simulink model "testing_discrete_tf"  (R2015b)
settings: Solver=ode23t  StartTime=0.0  StopTime=10.0  RelTol=1e-3
values from neighbouring files (symbols this model uses):
  tfa = dis_num_c2{1,1}(1)    [compensator_design.m]
  tfb = dis_num_c2{1,1}(2)    [compensator_design.m]
  tfc = dis_num_c2{1,1}(3)    [compensator_design.m]
  tfd = dis_den_c2{1,1}(1)    [compensator_design.m]
  tfe = dis_den_c2{1,1}(2)    [compensator_design.m]
  tff = dis_den_c2{1,1}(3)    [compensator_design.m]
undefined symbols (not defined in the file or in its folder): dis_den_c2, dis_num_c2
settings Model: Creator=Akshay  LastModifiedBy=Akshay

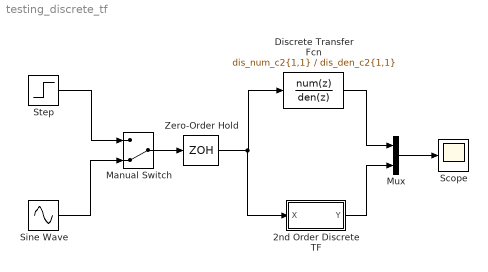
== system testing_discrete_tf ==
  2nd Order Discrete TF : Subsystem
  Discrete Transfer Fcn : DiscreteTransferFcn  Numerator=dis_num_c2{1,1}  Denominator=dis_den_c2{1,1}
  Manual Switch : ManualSwitch  CurrentSetting=0
  Mux : Mux  Inputs=2
  Scope : Scope
  Sine Wave : Sin  SampleTime=0
  Step : Step  SampleTime=0
  Zero-Order Hold : ZeroOrderHold  SampleTime=1e-5
  wires:
  Step/1 -> Manual Switch/1
  Sine Wave/1 -> Manual Switch/2
  Discrete Transfer Fcn/1 -> Mux/1
  2nd Order Discrete TF/1(Y) -> Mux/2
  Mux/1 -> Scope/1
  Manual Switch/1 -> Zero-Order Hold/1
  Zero-Order Hold/1 -> 2nd Order Discrete TF/1(X), Discrete Transfer Fcn/1

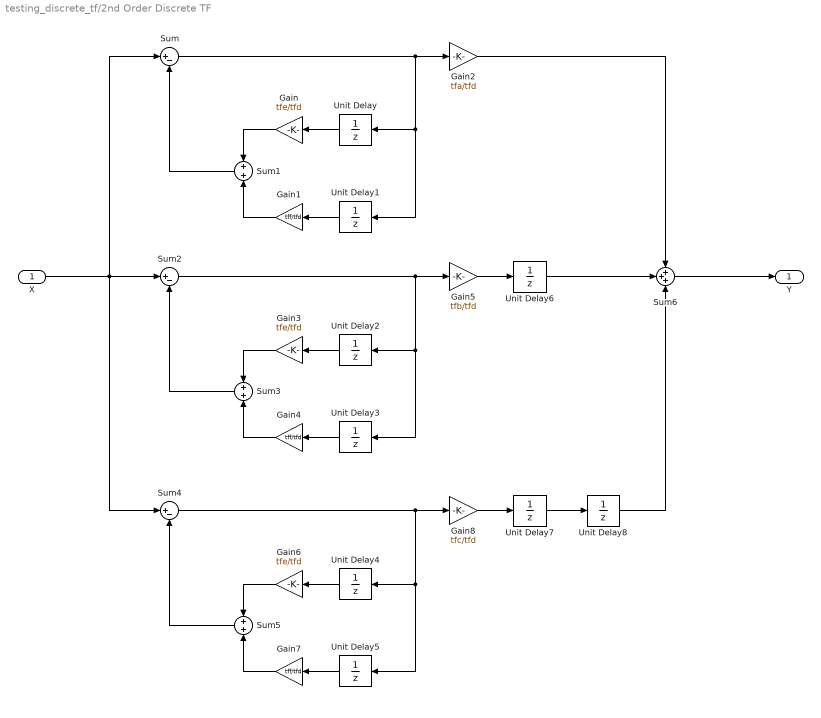
== system testing_discrete_tf/2nd Order Discrete TF ==
  X : Inport
  Gain : Gain  Gain=tfe/tfd
  Gain1 : Gain  Gain=tff/tfd
  Gain2 : Gain  Gain=tfa/tfd
  Gain3 : Gain  Gain=tfe/tfd
  Gain4 : Gain  Gain=tff/tfd
  Gain5 : Gain  Gain=tfb/tfd
  Gain6 : Gain  Gain=tfe/tfd
  Gain7 : Gain  Gain=tff/tfd
  Gain8 : Gain  Gain=tfc/tfd
  Sum : Sum  Inputs=|+-
  Sum1 : Sum
  Sum2 : Sum  Inputs=|+-
  Sum3 : Sum
  Sum4 : Sum  Inputs=|+-
  Sum5 : Sum
  Sum6 : Sum  Inputs=+++
  Unit Delay{,1..8} (9 alike) : UnitDelay  SampleTime=-1
  Y : Outport
  wires:
  Unit Delay/1 -> Gain/1
  Gain/1 -> Sum1/1
  Gain1/1 -> Sum1/2
  Unit Delay1/1 -> Gain1/1
  Sum1/1 -> Sum/2
  Sum/1 -> Gain2/1, Unit Delay1/1, Unit Delay/1
  Unit Delay6/1 -> Sum6/2
  Unit Delay3/1 -> Gain4/1
  Gain5/1 -> Unit Delay6/1
  X/1 -> Sum/1, Sum4/1, Sum2/1
  Sum2/1 -> Gain5/1, Unit Delay3/1, Unit Delay2/1
  Unit Delay2/1 -> Gain3/1
  Gain3/1 -> Sum3/1
  Gain4/1 -> Sum3/2
  Gain2/1 -> Sum6/1
  Sum3/1 -> Sum2/2
  Sum5/1 -> Sum4/2
  Sum4/1 -> Gain8/1, Unit Delay5/1, Unit Delay4/1
  Unit Delay7/1 -> Unit Delay8/1
  Gain7/1 -> Sum5/2
  Gain6/1 -> Sum5/1
  Unit Delay5/1 -> Gain7/1
  Gain8/1 -> Unit Delay7/1
  Unit Delay4/1 -> Gain6/1
  Sum6/1 -> Y/1
  Unit Delay8/1 -> Sum6/3
